simulink model "CruiseControl_PartialCoverageValid_harness"  (R2015a)
settings: Solver=FixedStepDiscrete  StartTime=0.0  StopTime=2  FixedStep=0.1  RelTol=1e-3
model workspace (MAT data in the model file):
  AccelResSw = mpt.Signal
  AccelResSw.DataType = 'boolean'
  AccelResSw.Min = 0
  AccelResSw.Max = 1
  AccelResSw.Dimensions = 1
  AccelResSw.DimensionsMode = 'Fixed'
  AccelResSw.Complexity = 'auto'
  AccelResSw.SampleTime = -1
  AccelResSw.SamplingMode = 'auto'
  Brake = mpt.Signal
  Brake.DataType = 'boolean'
  Brake.Min = 0
  Brake.Max = 1
  Brake.Dimensions = 1
  Brake.DimensionsMode = 'Fixed'
  Brake.Complexity = 'auto'
  Brake.SampleTime = -1
  Brake.SamplingMode = 'auto'
  CoastSetSw = mpt.Signal
  CoastSetSw.DataType = 'boolean'
  CoastSetSw.Min = 0
  CoastSetSw.Max = 1
  CoastSetSw.Dimensions = 1
  CoastSetSw.DimensionsMode = 'Fixed'
  CoastSetSw.Complexity = 'auto'
  CoastSetSw.SampleTime = -1
  CoastSetSw.SamplingMode = 'auto'
  CruiseOnOff = mpt.Signal
  CruiseOnOff.DataType = 'boolean'
  CruiseOnOff.Min = 0
  CruiseOnOff.Max = 1
  CruiseOnOff.Dimensions = 1
  CruiseOnOff.DimensionsMode = 'Fixed'
  CruiseOnOff.Complexity = 'auto'
  CruiseOnOff.SampleTime = -1
  CruiseOnOff.SamplingMode = 'auto'
  Speed = mpt.Signal
  Speed.DataType = 'uint8'
  Speed.Min = 0
  Speed.Max = 160
  Speed.Dimensions = 1
  Speed.DimensionsMode = 'Fixed'
  Speed.Complexity = 'auto'
  Speed.SampleTime = -1
  Speed.SamplingMode = 'auto'
  engaged = mpt.Signal
  engaged.DataType = 'boolean'
  engaged.Min = 0
  engaged.Max = 1
  engaged.Dimensions = 1
  engaged.DimensionsMode = 'Fixed'
  engaged.Complexity = 'auto'
  engaged.SampleTime = -1
  engaged.SamplingMode = 'auto'
  holdrate = mpt.Parameter
  holdrate.Value = 5
  holdrate.DataType = 'uint8'
  holdrate.Min = 1
  holdrate.Max = 10
  incdec = mpt.Parameter
  incdec.Value = 1
  incdec.DataType = 'uint8'
  incdec.Min = 1
  incdec.Max = 2
  maxtspeed = mpt.Parameter
  maxtspeed.Value = 90
  maxtspeed.DataType = 'uint8'
  maxtspeed.Min = 80
  maxtspeed.Max = 90
  mintspeed = mpt.Parameter
  mintspeed.Value = 20
  mintspeed.DataType = 'uint8'
  mintspeed.Min = 20
  mintspeed.Max = 25
  tspeed = mpt.Signal
  tspeed.DataType = 'uint8'
  tspeed.Min = 0
  tspeed.Max = 160
  tspeed.Dimensions = 1
  tspeed.DimensionsMode = 'Fixed'
  tspeed.Complexity = 'auto'
  tspeed.SampleTime = -1
  tspeed.SamplingMode = 'auto'
undefined symbols (not defined in the file or in its folder): sigbuilder_block
settings Model: PauseTimes=1.5  CovMetricSettings=dcmw  CovHTMLOptions=-sRT=1 -sVT=0 -aTS=0 -bRG=1 -bTC=1 -hTR=0 -nFC=0 -scm=1 -bcm=1 -xEv=0  CovSaveSingleToWorkspaceVar=off  CovCumulativeReport=on  CovReportOnPause=off  CovModelRefEnable=all  CovSFcnEnable=off  Creator=colosky  LastModifiedBy=colosky
settings DataIOCC: InspectSignalLogs=on
settings DebuggingCC: UnderspecifiedInitializationDetection=Classic  MergeDetectMultiDrivingBlocksExec=none  SolverPrmCheckMsg=warning

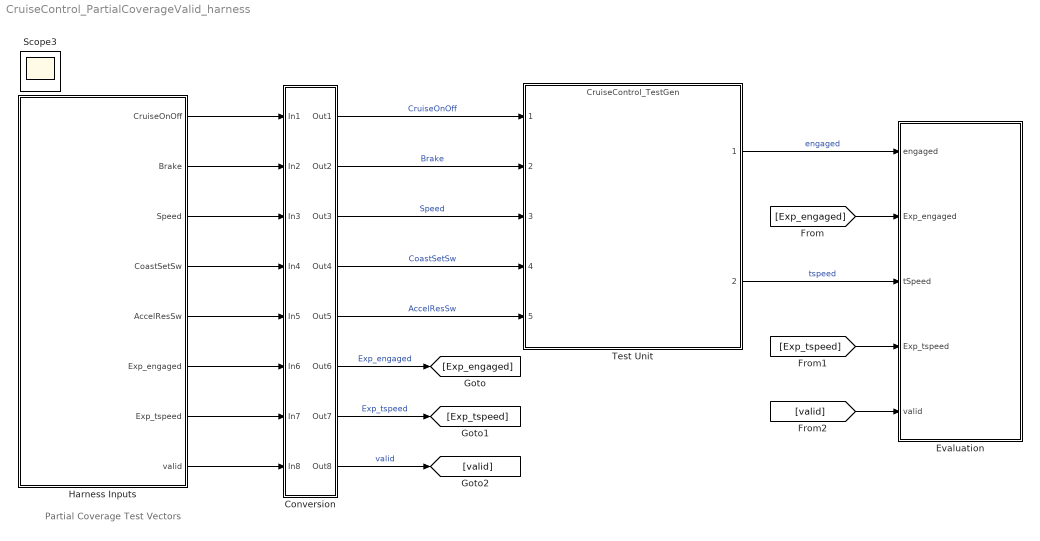
== system CruiseControl_PartialCoverageValid_harness ==
  note: Partial Coverage Test Vectors
  Conversion : Subsystem
      mask Display: disp(['Data' char(10) 'Type' char(10) 'Conv']);
  Evaluation : Subsystem
  Harness Inputs : Subsystem  Tag=STV Subsys  LoadFcn=sigbuilder_block('load',[756.6 77.4 520.2 400.2 ]);  StartFcn=sigbuilder_block('start');  StopFcn=sigbuilder_block('stop');  ClipboardFcn=sigbuilder_block('clipboard');  mask(Sigbuilder block){}
      mask init:
      | if ~strcmp(get_param(bdroot(gcb),'SimulationStatus'),'stopped'),tuvar = sigbuilder_block('maskInit'); end
      settings: CopyFcn=sigbuilder_block('copy');  DeleteFcn=sigbuilder_block('delete');  ModelCloseFcn=sigbuilder_block('modelClose');  PreSaveFcn=sigbuilder_block('preSave');  PauseFcn=sigbuilder_block('pause');  ContinueFcn=sigbuilder_block('continue');  NameChangeFcn=sigbuilder_block('namechange');  OpenFcn=sigbuilder_block('open');  CloseFcn=sigbuilder_block('close');
      mask Display: plot(0, 0, 100, 100,[2, 2, 32, 32, 2], [68, 8, 8, 68, 68],[32, 2], [38, 38], [32, 19, 2],[53, 60, 44], [32, 17, 17, 2],[16, 16, 31, 31]);txt = getActiveGroup(gcbh);text(2, 100, txt,'verticalAlignment', 'top');
  Test Unit : ModelReference  ModelNameDialog=CruiseControl_TestGen.slx  SimulationMode=Normal  ModelReferenceVersion=1.449  CopyOfModelName=CruiseControl_TestGen.slx  DefaultDataLogging=on
  Scope3 : Scope
      settings: SaveName=ScopeData3  MaxDataPoints=7500
  wires:
  Conversion/1(Out1) -> Test Unit/1  "CruiseOnOff"
  Conversion/5(Out5) -> Test Unit/5  "AccelResSw"
  Conversion/2(Out2) -> Test Unit/2  "Brake"
  Conversion/4(Out4) -> Test Unit/4  "CoastSetSw"
  Conversion/3(Out3) -> Test Unit/3  "Speed"
  Conversion/6(Out6) -> [Exp_engaged]  "Exp_engaged"
  Conversion/7(Out7) -> [Exp_tspeed]  "Exp_tspeed"
  Test Unit/1 -> Evaluation/1(engaged)  "engaged"
  Test Unit/2 -> Evaluation/3(tSpeed)  "tspeed"
  [Exp_engaged] -> Evaluation/2(Exp_engaged)
  [Exp_tspeed] -> Evaluation/4(Exp_tspeed)
  Harness Inputs/2(Brake) -> Conversion/2(In2)
  Harness Inputs/3(Speed) -> Conversion/3(In3)
  Harness Inputs/1(CruiseOnOff) -> Conversion/1(In1)
  Harness Inputs/4(CoastSetSw) -> Conversion/4(In4)
  Harness Inputs/5(AccelResSw) -> Conversion/5(In5)
  Harness Inputs/6(Exp_engaged) -> Conversion/6(In6)
  Harness Inputs/7(Exp_tspeed) -> Conversion/7(In7)
  Harness Inputs/8(valid) -> Conversion/8(In8)
  Conversion/8(Out8) -> [valid]  "valid"
  [valid] -> Evaluation/5(valid)

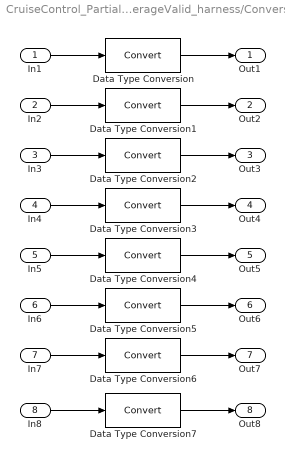
== system CruiseControl_PartialCoverageValid_harness/Conversion ==
  In1 : Inport
  In2 : Inport  Port=2
  In3 : Inport  Port=3
  In4 : Inport  Port=4
  In5 : Inport  Port=5
  In6 : Inport  Port=6
  In7 : Inport  Port=7
  In8 : Inport  Port=8
  Data Type Conversion{,1..7} (8 alike) : DataTypeConversion
  Out1 : Outport
  Out2 : Outport  Port=2
  Out3 : Outport  Port=3
  Out4 : Outport  Port=4
  Out5 : Outport  Port=5
  Out6 : Outport  Port=6
  Out7 : Outport  Port=7
  Out8 : Outport  Port=8
  wires:
  Data Type Conversion7/1 -> Out8/1
  In8/1 -> Data Type Conversion7/1
  In4/1 -> Data Type Conversion3/1
  Data Type Conversion4/1 -> Out5/1
  Data Type Conversion1/1 -> Out2/1
  In1/1 -> Data Type Conversion/1
  Data Type Conversion/1 -> Out1/1
  Data Type Conversion5/1 -> Out6/1
  In6/1 -> Data Type Conversion5/1
  Data Type Conversion6/1 -> Out7/1
  In7/1 -> Data Type Conversion6/1
  In5/1 -> Data Type Conversion4/1
  In2/1 -> Data Type Conversion1/1
  Data Type Conversion3/1 -> Out4/1
  In3/1 -> Data Type Conversion2/1
  Data Type Conversion2/1 -> Out3/1

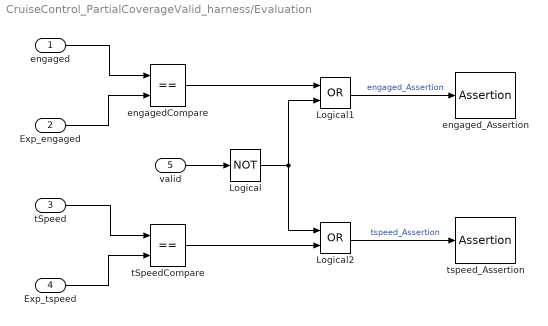
== system CruiseControl_PartialCoverageValid_harness/Evaluation ==
  engaged : Inport
  Exp_engaged : Inport  Port=2
  tSpeed : Inport  Port=3
  Exp_tspeed : Inport  Port=4
  valid : Inport  Port=5
  Logical : Logic  Operator=NOT  OutDataTypeStr=boolean
  Logical1 : Logic  Operator=OR  OutDataTypeStr=boolean
  Logical2 : Logic  Operator=OR  OutDataTypeStr=boolean
  engagedCompare : RelationalOperator  Operator===  OutDataTypeStr=boolean  InputSameDT=on
  engaged_Assertion : Assertion
  tSpeedCompare : RelationalOperator  Operator===  OutDataTypeStr=boolean  InputSameDT=on
  tspeed_Assertion : Assertion
  wires:
  Exp_engaged/1 -> engagedCompare/2
  engaged/1 -> engagedCompare/1
  Exp_tspeed/1 -> tSpeedCompare/2
  tSpeed/1 -> tSpeedCompare/1
  engagedCompare/1 -> Logical1/1
  tSpeedCompare/1 -> Logical2/2
  valid/1 -> Logical/1
  Logical1/1 -> engaged_Assertion/1  "engaged_Assertion"
  Logical/1 -> Logical2/1, Logical1/2
  Logical2/1 -> tspeed_Assertion/1  "tspeed_Assertion"

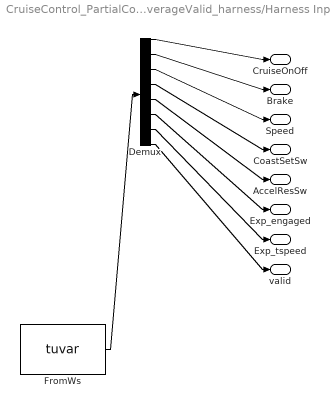
== system CruiseControl_PartialCoverageValid_harness/Harness Inputs ==
  Demux : Demux  Tag=STV Demux  Outputs=8
  FromWs : FromWorkspace  Tag=STV FromWs  VariableName=tuvar  SampleTime=0
      SigBuilderData=|
      | dataSet(1).timeRange = [0 2]
      | dataSet(1).name = 'Init Not Enable or Engaged'
      | dataSet(2).timeRange = [0 2]
      | dataSet(2).name = 'Not Engaged with Enable'
      | dataSet(3).timeRange = [0 2]
      | dataSet(3).name = 'Disengage with Disable'
      | dataSet(4).timeRange = [0 2]
      | dataSet(4).name = 'Engage 1st with CoastSetSW'
      | dataSet(5).timeRange = [0 2]
      | dataSet(5).name = 'No Engage 1st with AccelResSW'
      | dataSet(6).timeRange = [0 2]
      | dataSet(6).name = 'Disengage with Brake'
      | dataSet(7).timeRange = [0 2]
      | dataSet(7).name = 'Re-Engage with CoastSetSw'
      | dataSet(8).timeRange = [0 2]
      | dataSet(8).name = 'Re-Engage with AccelResSw'
      | dataSet(9).timeRange = [0 2]
      | dataSet(9).name = 'Engaged Decel with CoastSetSW'
      | dataSet(10).timeRange = [0 2]
      | dataSet(10).name = 'Engaged Accel with AccelResSW '
      | dataSet(11).timeRange = [0 2]
      | dataSet(11).name = 'Engagd Decel with CoastSet Hold'
      | dataSet(12).timeRange = [0 2]
      | dataSet(12).name = 'Engagd Accel with AccelRes Hold'
      | dataSet(13).timeRange = [0 2]
      | dataSet(13).name = 'Engage CoastSetSw Veh Spd'
      | dataSet(14).timeRange = [0 2]
      | dataSet(14).name = 'Engage AccelResSw Veh Spd '
      | sbobj.Name = 'Signal Builder'
      | sbobj.Groups(1).Name = 'Init Not Enable or Engaged'
      | sbobj.Groups(1).Signals(1).Name = 'CruiseOnOff'
      | sbobj.Groups(1).Signals(1).XData = [0 1 2]
      | sbobj.Groups(1).Signals(1).YData = [0 0 0]
      | sbobj.Groups(1).Signals(2).Name = 'Brake'
      | sbobj.Groups(1).Signals(2).XData = [0 1 2]
      | sbobj.Groups(1).Signals(2).YData = [0 0 0]
      | sbobj.Groups(1).Signals(3).Name = 'Speed'
      | sbobj.Groups(1).Signals(3).XData = [0 1 2]
      | sbobj.Groups(1).Signals(3).YData = [50 50 50]
      | sbobj.Groups(1).Signals(4).Name = 'CoastSetSw'
      | sbobj.Groups(1).Signals(4).XData = [0 1 2]
      | sbobj.Groups(1).Signals(4).YData = [0 0 0]
      | sbobj.Groups(1).Signals(5).Name = 'AccelResSw'
      | sbobj.Groups(1).Signals(5).XData = [0 1 2]
      | sbobj.Groups(1).Signals(5).YData = [0 0 0]
      | sbobj.Groups(1).Signals(6).Name = 'Exp_engaged'
      | sbobj.Groups(1).Signals(6).XData = [0 1 2]
      | sbobj.Groups(1).Signals(6).YData = [0 0 0]
      | sbobj.Groups(1).Signals(7).Name = 'Exp_tspeed'
      | sbobj.Groups(1).Signals(7).XData = [0 1 2]
      | sbobj.Groups(1).Signals(7).YData = [0 0 0]
      | sbobj.Groups(1).Signals(8).Name = 'valid'
      | sbobj.Groups(1).Signals(8).XData = [0 2]
      | sbobj.Groups(1).Signals(8).YData = [1 1]
      | sbobj.Groups(1).TimeRange = [0 2]
      | sbobj.Groups(2).Name = 'Not Engaged with Enable'
      | sbobj.Groups(2).Signals(1).Name = 'CruiseOnOff'
      | sbobj.Groups(2).Signals(1).XData = [0 1 1 1.5 1.5 2]
      | sbobj.Groups(2).Signals(1).YData = [0 0 1 1 0 0]
      | sbobj.Groups(2).Signals(2).Name = 'Brake'
      | sbobj.Groups(2).Signals(2).XData = [0 1 1.5 2]
      | sbobj.Groups(2).Signals(2).YData = [0 0 0 0]
      | sbobj.Groups(2).Signals(3).Name = 'Speed'
      | sbobj.Groups(2).Signals(3).XData = [0 1 1.5 2]
      | sbobj.Groups(2).Signals(3).YData = [0 0 0 0]
      | sbobj.Groups(2).Signals(4).Name = 'CoastSetSw'
      | sbobj.Groups(2).Signals(4).XData = [0 1 1.5 2]
      | sbobj.Groups(2).Signals(4).YData = [0 0 0 0]
      | sbobj.Groups(2).Signals(5).Name = 'AccelResSw'
      | sbobj.Groups(2).Signals(5).XData = [0 1 1.5 2]
      | sbobj.Groups(2).Signals(5).YData = [0 0 0 0]
      | sbobj.Groups(2).Signals(6).Name = 'Exp_engaged'
      | sbobj.Groups(2).Signals(6).XData = [0 1 1.5 2]
      | sbobj.Groups(2).Signals(6).YData = [0 0 0 0]
      | sbobj.Groups(2).Signals(7).Name = 'Exp_tspeed'
      | sbobj.Groups(2).Signals(7).XData = [0 1 1.5 2]
      | sbobj.Groups(2).Signals(7).YData = [0 0 0 0]
      | sbobj.Groups(2).Signals(8).Name = 'valid'
      | sbobj.Groups(2).Signals(8).XData = [0 2]
      | sbobj.Groups(2).Signals(8).YData = [1 1]
      | sbobj.Groups(2).TimeRange = [0 2]
      | sbobj.Groups(3).Name = 'Disengage with Disable'
      | sbobj.Groups(3).Signals(1).Name = 'CruiseOnOff'
      | sbobj.Groups(3).Signals(1).XData = [0 0.5 0.5 1 1.1 1.5 1.5 2]
      | sbobj.Groups(3).Signals(1).YData = [0 0 1 1 1 1 0 0]
      | sbobj.Groups(3).Signals(2).Name = 'Brake'
      | sbobj.Groups(3).Signals(2).XData = [0 0.5 1 1.1 1.5 2]
      | sbobj.Groups(3).Signals(2).YData = [0 0 0 0 0 0]
      | sbobj.Groups(3).Signals(3).Name = 'Speed'
      | sbobj.Groups(3).Signals(3).XData = [0 0.5 1 1.1 1.5 2]
      | sbobj.Groups(3).Signals(3).YData = [50 50 50 50 50 50]
      | sbobj.Groups(3).Signals(4).Name = 'CoastSetSw'
      | sbobj.Groups(3).Signals(4).XData = [0 0.5 1 1 1.1 1.1 1.5 2]
      | sbobj.Groups(3).Signals(4).YData = [0 0 0 1 1 0 0 0]
      | sbobj.Groups(3).Signals(5).Name = 'AccelResSw'
      | sbobj.Groups(3).Signals(5).XData = [0 0.5 1 1.1 1.5 2]
      | sbobj.Groups(3).Signals(5).YData = [0 0 0 0 0 0]
      | sbobj.Groups(3).Signals(6).Name = 'Exp_engaged'
      | sbobj.Groups(3).Signals(6).XData = [0 0.5 1 1 1.1 1.5 1.5 2]
      | sbobj.Groups(3).Signals(6).YData = [0 0 0 1 1 1 0 0]
      | sbobj.Groups(3).Signals(7).Name = 'Exp_tspeed'
      | sbobj.Groups(3).Signals(7).XData = [0 0.5 1 1 1.1 1.5 1.5 2]
      | sbobj.Groups(3).Signals(7).YData = [0 0 0 50 50 50 0 0]
      | sbobj.Groups(3).Signals(8).Name = 'valid'
      | sbobj.Groups(3).Signals(8).XData = [0 2]
      | sbobj.Groups(3).Signals(8).YData = [1 1]
      | sbobj.Groups(3).TimeRange = [0 2]
      | sbobj.Groups(4).Name = 'Engage 1st with CoastSetSW'
      | sbobj.Groups(4).Signals(1).Name = 'CruiseOnOff'
      | sbobj.Groups(4).Signals(1).XData = [0 0.5 0.5 1 1.1 2]
      | sbobj.Groups(4).Signals(1).YData = [0 0 1 1 1 1]
      | sbobj.Groups(4).Signals(2).Name = 'Brake'
      | sbobj.Groups(4).Signals(2).XData = [0 0.5 1 1.1 2]
      | sbobj.Groups(4).Signals(2).YData = [0 0 0 0 0]
      | sbobj.Groups(4).Signals(3).Name = 'Speed'
      | sbobj.Groups(4).Signals(3).XData = [0 0.5 1 1.1 2]
      | sbobj.Groups(4).Signals(3).YData = [50 50 50 50 50]
      | sbobj.Groups(4).Signals(4).Name = 'CoastSetSw'
      | sbobj.Groups(4).Signals(4).XData = [0 0.5 1 1 1.1 1.1 2]
      | sbobj.Groups(4).Signals(4).YData = [0 0 0 1 1 0 0]
      | sbobj.Groups(4).Signals(5).Name = 'AccelResSw'
      | sbobj.Groups(4).Signals(5).XData = [0 0.5 1 1.1 2]
      | sbobj.Groups(4).Signals(5).YData = [0 0 0 0 0]
      | sbobj.Groups(4).Signals(6).Name = 'Exp_engaged'
      | sbobj.Groups(4).Signals(6).XData = [0 0.5 1 1 1.1 2]
      | sbobj.Groups(4).Signals(6).YData = [0 0 0 1 1 1]
      | sbobj.Groups(4).Signals(7).Name = 'Exp_tspeed'
      | sbobj.Groups(4).Signals(7).XData = [0 0.5 1 1 1.1 2]
      | sbobj.Groups(4).Signals(7).YData = [0 0 0 50 50 50]
      | sbobj.Groups(4).Signals(8).Name = 'valid'
      | sbobj.Groups(4).Signals(8).XData = [0 2]
      | sbobj.Groups(4).Signals(8).YData = [1 1]
      | sbobj.Groups(4).TimeRange = [0 2]
      | sbobj.Groups(5).Name = 'No Engage 1st with AccelResSW'
      | sbobj.Groups(5).Signals(1).Name = 'CruiseOnOff'
      | sbobj.Groups(5).Signals(1).XData = [0 0.5 0.5 1 1.1 2]
      | sbobj.Groups(5).Signals(1).YData = [0 0 1 1 1 1]
      | sbobj.Groups(5).Signals(2).Name = 'Brake'
      | sbobj.Groups(5).Signals(2).XData = [0 0.5 1 1.1 2]
      | sbobj.Groups(5).Signals(2).YData = [0 0 0 0 0]
      | sbobj.Groups(5).Signals(3).Name = 'Speed'
      | sbobj.Groups(5).Signals(3).XData = [0 0.5 1 1.1 2]
      | sbobj.Groups(5).Signals(3).YData = [50 50 50 50 50]
      | sbobj.Groups(5).Signals(4).Name = 'CoastSetSw'
      | sbobj.Groups(5).Signals(4).XData = [0 0.5 1 1.1 2]
      | sbobj.Groups(5).Signals(4).YData = [0 0 0 0 0]
      | sbobj.Groups(5).Signals(5).Name = 'AccelResSw'
      | sbobj.Groups(5).Signals(5).XData = [0 0.5 1 1 1.1 1.1 2]
      | sbobj.Groups(5).Signals(5).YData = [0 0 0 1 1 0 0]
      | sbobj.Groups(5).Signals(6).Name = 'Exp_engaged'
      | sbobj.Groups(5).Signals(6).XData = [0 0.5 1 1.1 2]
      | sbobj.Groups(5).Signals(6).YData = [0 0 0 0 0]
      | sbobj.Groups(5).Signals(7).Name = 'Exp_tspeed'
      | sbobj.Groups(5).Signals(7).XData = [0 0.5 1 1.1 2]
      | sbobj.Groups(5).Signals(7).YData = [0 0 0 0 0]
      | sbobj.Groups(5).Signals(8).Name = 'valid'
      | sbobj.Groups(5).Signals(8).XData = [0 2]
      | sbobj.Groups(5).Signals(8).YData = [1 1]
      | sbobj.Groups(5).TimeRange = [0 2]
      | sbobj.Groups(6).Name = 'Disengage with Brake'
      | sbobj.Groups(6).Signals(1).Name = 'CruiseOnOff'
      | sbobj.Groups(6).Signals(1).XData = [0 0.5 0.5 1 1.1 1.5 1.6 2]
      | sbobj.Groups(6).Signals(1).YData = [0 0 1 1 1 1 1 1]
      | sbobj.Groups(6).Signals(2).Name = 'Brake'
      | sbobj.Groups(6).Signals(2).XData = [0 0.5 1 1.1 1.5 1.5 1.6 1.6 2]
      | sbobj.Groups(6).Signals(2).YData = [0 0 0 0 0 1 1 0 0]
      | sbobj.Groups(6).Signals(3).Name = 'Speed'
      | sbobj.Groups(6).Signals(3).XData = [0 0.5 1 1.1 1.5 1.6 2]
      | sbobj.Groups(6).Signals(3).YData = [50 50 50 50 50 50 50]
      | sbobj.Groups(6).Signals(4).Name = 'CoastSetSw'
      | sbobj.Groups(6).Signals(4).XData = [0 0.5 1 1 1.1 1.1 1.5 1.6 2]
      | sbobj.Groups(6).Signals(4).YData = [0 0 0 1 1 0 0 0 0]
      | sbobj.Groups(6).Signals(5).Name = 'AccelResSw'
      | sbobj.Groups(6).Signals(5).XData = [0 0.5 1 1.1 1.5 1.6 2]
      | sbobj.Groups(6).Signals(5).YData = [0 0 0 0 0 0 0]
      | sbobj.Groups(6).Signals(6).Name = 'Exp_engaged'
      | sbobj.Groups(6).Signals(6).XData = [0 0.5 1 1 1.1 1.5 1.5 1.6 2]
      | sbobj.Groups(6).Signals(6).YData = [0 0 0 1 1 1 0 0 0]
      | sbobj.Groups(6).Signals(7).Name = 'Exp_tspeed'
      | sbobj.Groups(6).Signals(7).XData = [0 0.5 1 1 1.1 1.5 1.6 2]
      | sbobj.Groups(6).Signals(7).YData = [0 0 0 50 50 50 50 50]
      | sbobj.Groups(6).Signals(8).Name = 'valid'
      | sbobj.Groups(6).Signals(8).XData = [0 2]
      | sbobj.Groups(6).Signals(8).YData = [1 1]
      | sbobj.Groups(6).TimeRange = [0 2]
      | sbobj.Groups(7).Name = 'Re-Engage with CoastSetSw'
      | sbobj.Groups(7).Signals(1).Name = 'CruiseOnOff'
      | sbobj.Groups(7).Signals(1).XData = [0 0.5 0.5 1 1.1 1.3 1.5 1.7 1.8 2]
      | sbobj.Groups(7).Signals(1).YData = [0 0 1 1 1 1 1 1 1 1]
      | sbobj.Groups(7).Signals(2).Name = 'Brake'
      | sbobj.Groups(7).Signals(2).XData = [0 0.5 1 1.1 1.3 1.3 1.5 1.5 1.7 1.8 2]
      | sbobj.Groups(7).Signals(2).YData = [0 0 0 0 0 1 1 0 0 0 0]
      | sbobj.Groups(7).Signals(3).Name = 'Speed'
      | sbobj.Groups(7).Signals(3).XData = [0 0.5 1 1.1 1.3 1.5 1.7 1.7 1.8 2]
      | sbobj.Groups(7).Signals(3).YData = [50 50 50 50 50 50 50 60 60 60]
      | sbobj.Groups(7).Signals(4).Name = 'CoastSetSw'
      | sbobj.Groups(7).Signals(4).XData = [0 0.5 1 1 1.1 1.1 1.3 1.5 1.7 1.7 1.8 1.8 2]
      | sbobj.Groups(7).Signals(4).YData = [0 0 0 1 1 0 0 0 0 1 1 0 0]
      | sbobj.Groups(7).Signals(5).Name = 'AccelResSw'
      | sbobj.Groups(7).Signals(5).XData = [0 0.5 1 1.1 1.3 1.5 1.7 1.8 2]
      | sbobj.Groups(7).Signals(5).YData = [0 0 0 0 0 0 0 0 0]
      | sbobj.Groups(7).Signals(6).Name = 'Exp_engaged'
      | sbobj.Groups(7).Signals(6).XData = [0 0.5 1 1 1.1 1.3 1.3 1.5 1.7 1.7 1.8 2]
      | sbobj.Groups(7).Signals(6).YData = [0 0 0 1 1 1 0 0 0 1 1 1]
      | sbobj.Groups(7).Signals(7).Name = 'Exp_tspeed'
      | sbobj.Groups(7).Signals(7).XData = [0 0.5 1 1 1.1 1.3 1.5 1.7 1.7 1.8 2]
      | sbobj.Groups(7).Signals(7).YData = [0 0 0 50 50 50 50 50 60 60 60]
      | sbobj.Groups(7).Signals(8).Name = 'valid'
      | sbobj.Groups(7).Signals(8).XData = [0 2]
      | sbobj.Groups(7).Signals(8).YData = [1 1]
      | sbobj.Groups(7).TimeRange = [0 2]
      | sbobj.Groups(8).Name = 'Re-Engage with AccelResSw'
      | sbobj.Groups(8).Signals(1).Name = 'CruiseOnOff'
      | sbobj.Groups(8).Signals(1).XData = [0 0.5 0.5 1 1.1 1.3 1.5 1.7 1.8 2]
      | sbobj.Groups(8).Signals(1).YData = [0 0 1 1 1 1 1 1 1 1]
      | sbobj.Groups(8).Signals(2).Name = 'Brake'
      | sbobj.Groups(8).Signals(2).XData = [0 0.5 1 1.1 1.3 1.3 1.5 1.5 1.7 1.8 2]
      | sbobj.Groups(8).Signals(2).YData = [0 0 0 0 0 1 1 0 0 0 0]
      | sbobj.Groups(8).Signals(3).Name = 'Speed'
      | sbobj.Groups(8).Signals(3).XData = [0 0.5 1 1.1 1.3 1.5 1.7 1.7 1.8 2]
      | sbobj.Groups(8).Signals(3).YData = [50 50 50 50 50 50 50 60 60 60]
      | sbobj.Groups(8).Signals(4).Name = 'CoastSetSw'
      | sbobj.Groups(8).Signals(4).XData = [0 0.5 1 1 1.1 1.1 1.3 1.5 1.7 1.8 2]
      | sbobj.Groups(8).Signals(4).YData = [0 0 0 1 1 0 0 0 0 0 0]
      | sbobj.Groups(8).Signals(5).Name = 'AccelResSw'
      | sbobj.Groups(8).Signals(5).XData = [0 0.5 1 1.1 1.3 1.5 1.7 1.7 1.8 1.8 2]
      | sbobj.Groups(8).Signals(5).YData = [0 0 0 0 0 0 0 1 1 0 0]
      | sbobj.Groups(8).Signals(6).Name = 'Exp_engaged'
      | sbobj.Groups(8).Signals(6).XData = [0 0.5 1 1 1.1 1.3 1.3 1.5 1.7 1.7 1.8 2]
      | sbobj.Groups(8).Signals(6).YData = [0 0 0 1 1 1 0 0 0 1 1 1]
      | sbobj.Groups(8).Signals(7).Name = 'Exp_tspeed'
      | sbobj.Groups(8).Signals(7).XData = [0 0.5 1 1 1.1 1.3 1.5 1.7 1.8 2]
      | sbobj.Groups(8).Signals(7).YData = [0 0 0 50 50 50 50 50 50 50]
      | sbobj.Groups(8).Signals(8).Name = 'valid'
      | sbobj.Groups(8).Signals(8).XData = [0 2]
      | sbobj.Groups(8).Signals(8).YData = [1 1]
      | sbobj.Groups(8).TimeRange = [0 2]
      | sbobj.Groups(9).Name = 'Engaged Decel with CoastSetSW'
      | sbobj.Groups(9).Signals(1).Name = 'CruiseOnOff'
      | sbobj.Groups(9).Signals(1).XData = [0 0.5 0.5 1 1.1 1.5 1.6 1.7 1.8 2]
      | sbobj.Groups(9).Signals(1).YData = [0 0 1 1 1 1 1 1 1 1]
      | sbobj.Groups(9).Signals(2).Name = 'Brake'
      | sbobj.Groups(9).Signals(2).XData = [0 0.5 1 1.1 1.5 1.6 1.7 1.8 2]
      | sbobj.Groups(9).Signals(2).YData = [0 0 0 0 0 0 0 0 0]
      | sbobj.Groups(9).Signals(3).Name = 'Speed'
      | sbobj.Groups(9).Signals(3).XData = [0 0.5 1 1.1 1.5 1.6 1.7 1.8 2]
      | sbobj.Groups(9).Signals(3).YData = [50 50 50 50 50 50 50 50 50]
      | sbobj.Groups(9).Signals(4).Name = 'CoastSetSw'
      | sbobj.Groups(9).Signals(4).XData = [0 0.5 1 1 1.1 1.1 1.5 1.5 1.6 1.6 1.7 1.7 1.8 1.8 2]
      | sbobj.Groups(9).Signals(4).YData = [0 0 0 1 1 0 0 1 1 0 0 1 1 0 0]
      | sbobj.Groups(9).Signals(5).Name = 'AccelResSw'
      | sbobj.Groups(9).Signals(5).XData = [0 0.5 1 1.1 1.5 1.6 1.7 1.8 2]
      | sbobj.Groups(9).Signals(5).YData = [0 0 0 0 0 0 0 0 0]
      | sbobj.Groups(9).Signals(6).Name = 'Exp_engaged'
      | sbobj.Groups(9).Signals(6).XData = [0 0.5 1 1 1.1 1.5 1.6 1.7 1.8 2]
      | sbobj.Groups(9).Signals(6).YData = [0 0 0 1 1 1 1 1 1 1]
      | sbobj.Groups(9).Signals(7).Name = 'Exp_tspeed'
      | sbobj.Groups(9).Signals(7).XData = [0 0.5 1 1 1.1 1.5 1.5 1.6 1.7 1.7 1.8 2]
      | sbobj.Groups(9).Signals(7).YData = [0 0 0 50 50 50 49 49 49 48 48 48]
      | sbobj.Groups(9).Signals(8).Name = 'valid'
      | sbobj.Groups(9).Signals(8).XData = [0 2]
      | sbobj.Groups(9).Signals(8).YData = [1 1]
      | sbobj.Groups(9).TimeRange = [0 2]
      | sbobj.Groups(10).Name = 'Engaged Accel with AccelResSW '
      | sbobj.Groups(10).Signals(1).Name = 'CruiseOnOff'
      | sbobj.Groups(10).Signals(1).XData = [0 0.5 0.5 1 1.1 1.5 1.6 1.7 1.8 2]
      | sbobj.Groups(10).Signals(1).YData = [0 0 1 1 1 1 1 1 1 1]
      | sbobj.Groups(10).Signals(2).Name = 'Brake'
      | sbobj.Groups(10).Signals(2).XData = [0 0.5 1 1.1 1.5 1.6 1.7 1.8 2]
      | sbobj.Groups(10).Signals(2).YData = [0 0 0 0 0 0 0 0 0]
      | sbobj.Groups(10).Signals(3).Name = 'Speed'
      | sbobj.Groups(10).Signals(3).XData = [0 0.5 1 1.1 1.5 1.6 1.7 1.8 2]
      | sbobj.Groups(10).Signals(3).YData = [50 50 50 50 50 50 50 50 50]
      | sbobj.Groups(10).Signals(4).Name = 'CoastSetSw'
      | sbobj.Groups(10).Signals(4).XData = [0 0.5 1 1 1.1 1.1 1.5 1.6 1.7 1.8 2]
      | sbobj.Groups(10).Signals(4).YData = [0 0 0 1 1 0 0 0 0 0 0]
      | sbobj.Groups(10).Signals(5).Name = 'AccelResSw'
      | sbobj.Groups(10).Signals(5).XData = [0 0.5 1 1.1 1.5 1.5 1.6 1.6 1.7 1.7 1.8 1.8 2]
      | sbobj.Groups(10).Signals(5).YData = [0 0 0 0 0 1 1 0 0 1 1 0 0]
      | sbobj.Groups(10).Signals(6).Name = 'Exp_engaged'
      | sbobj.Groups(10).Signals(6).XData = [0 0.5 1 1 1.1 1.5 1.6 1.7 1.8 2]
      | sbobj.Groups(10).Signals(6).YData = [0 0 0 1 1 1 1 1 1 1]
      | sbobj.Groups(10).Signals(7).Name = 'Exp_tspeed'
      | sbobj.Groups(10).Signals(7).XData = [0 0.5 1 1 1.1 1.5 1.5 1.6 1.7 1.7 1.8 2]
      | sbobj.Groups(10).Signals(7).YData = [0 0 0 50 50 50 51 51 51 52 52 52]
      | sbobj.Groups(10).Signals(8).Name = 'valid'
      | sbobj.Groups(10).Signals(8).XData = [0 2]
      | sbobj.Groups(10).Signals(8).YData = [1 1]
      | sbobj.Groups(10).TimeRange = [0 2]
      | sbobj.Groups(11).Name = 'Engagd Decel with CoastSet Hold'
      | sbobj.Groups(11).Signals(1).Name = 'CruiseOnOff'
      | sbobj.Groups(11).Signals(1).XData = [0 0.2 0.2 0.5 0.6 1 1.1 1.3 1.5 1.7 1.8 2]
      | sbobj.Groups(11).Signals(1).YData = [0 0 1 1 1 1 1 1 1 1 1 1]
      | sbobj.Groups(11).Signals(2).Name = 'Brake'
      | sbobj.Groups(11).Signals(2).XData = [0 0.2 0.5 0.6 1 1.1 1.3 1.5 1.7 1.8 2]
      | sbobj.Groups(11).Signals(2).YData = [0 0 0 0 0 0 0 0 0 0 0]
      | sbobj.Groups(11).Signals(3).Name = 'Speed'
      | sbobj.Groups(11).Signals(3).XData = [0 0.2 0.5 0.6 0.6 1 1.1 1.3 1.5 1.7 1.8 2]
      | sbobj.Groups(11).Signals(3).YData = [50 50 50 50 40 40 40 40 40 40 40 40]
      | sbobj.Groups(11).Signals(4).Name = 'CoastSetSw'
      | sbobj.Groups(11).Signals(4).XData = [0 0.2 0.5 0.5 0.6 0.6 1 1 1.1 1.1 1.3 1.3 1.5 1.7 1.8 1.8 2]
      | sbobj.Groups(11).Signals(4).YData = [0 0 0 1 1 0 0 1 1 0 0 1 1 1 1 0 0]
      | sbobj.Groups(11).Signals(5).Name = 'AccelResSw'
      | sbobj.Groups(11).Signals(5).XData = [0 0.2 0.5 0.6 1 1.1 1.3 1.5 1.7 1.8 2]
      | sbobj.Groups(11).Signals(5).YData = [0 0 0 0 0 0 0 0 0 0 0]
      | sbobj.Groups(11).Signals(6).Name = 'Exp_engaged'
      | sbobj.Groups(11).Signals(6).XData = [0 0.2 0.5 0.5 0.6 1 1.1 1.3 1.5 1.7 1.8 2]
      | sbobj.Groups(11).Signals(6).YData = [0 0 0 1 1 1 1 1 1 1 1 1]
      | sbobj.Groups(11).Signals(7).Name = 'Exp_tspeed'
      | sbobj.Groups(11).Signals(7).XData = [0 0.2 0.5 0.5 0.6 1 1 1.1 1.3 1.3 1.5 1.5 1.7 1.7 1.8 2]
      | sbobj.Groups(11).Signals(7).YData = [0 0 0 50 50 50 49 49 49 48 48 47 47 46 46 46]
      | sbobj.Groups(11).Signals(8).Name = 'valid'
      | sbobj.Groups(11).Signals(8).XData = [0 2]
      | sbobj.Groups(11).Signals(8).YData = [1 1]
      | sbobj.Groups(11).TimeRange = [0 2]
      | sbobj.Groups(12).Name = 'Engagd Accel with AccelRes Hold'
      | sbobj.Groups(12).Signals(1).Name = 'CruiseOnOff'
      | sbobj.Groups(12).Signals(1).XData = [0 0.2 0.2 0.5 0.6 1 1.1 1.3 1.5 1.7 1.8 2]
      | sbobj.Groups(12).Signals(1).YData = [0 0 1 1 1 1 1 1 1 1 1 1]
      | sbobj.Groups(12).Signals(2).Name = 'Brake'
      | sbobj.Groups(12).Signals(2).XData = [0 0.2 0.5 0.6 1 1.1 1.3 1.5 1.7 1.8 2]
      | sbobj.Groups(12).Signals(2).YData = [0 0 0 0 0 0 0 0 0 0 0]
      | sbobj.Groups(12).Signals(3).Name = 'Speed'
      | sbobj.Groups(12).Signals(3).XData = [0 0.2 0.5 0.6 0.6 1 1.1 1.3 1.5 1.7 1.8 2]
      | sbobj.Groups(12).Signals(3).YData = [50 50 50 50 40 40 40 40 40 40 40 40]
      | sbobj.Groups(12).Signals(4).Name = 'CoastSetSw'
      | sbobj.Groups(12).Signals(4).XData = [0 0.2 0.5 0.5 0.6 0.6 1 1.1 1.3 1.5 1.7 1.8 2]
      | sbobj.Groups(12).Signals(4).YData = [0 0 0 1 1 0 0 0 0 0 0 0 0]
      | sbobj.Groups(12).Signals(5).Name = 'AccelResSw'
      | sbobj.Groups(12).Signals(5).XData = [0 0.2 0.5 0.6 1 1 1.1 1.1 1.3 1.3 1.5 1.7 1.8 1.8 2]
      | sbobj.Groups(12).Signals(5).YData = [0 0 0 0 0 1 1 0 0 1 1 1 1 0 0]
      | sbobj.Groups(12).Signals(6).Name = 'Exp_engaged'
      | sbobj.Groups(12).Signals(6).XData = [0 0.2 0.5 0.5 0.6 1 1.1 1.3 1.5 1.7 1.8 2]
      | sbobj.Groups(12).Signals(6).YData = [0 0 0 1 1 1 1 1 1 1 1 1]
      | sbobj.Groups(12).Signals(7).Name = 'Exp_tspeed'
      | sbobj.Groups(12).Signals(7).XData = [0 0.2 0.5 0.5 0.6 1 1 1.1 1.3 1.3 1.5 1.5 1.7 1.7 1.8 2]
      | sbobj.Groups(12).Signals(7).YData = [0 0 0 50 50 50 51 51 51 52 52 53 53 54 54 54]
      | sbobj.Groups(12).Signals(8).Name = 'valid'
      | sbobj.Groups(12).Signals(8).XData = [0 2]
      | sbobj.Groups(12).Signals(8).YData = [1 1]
      | sbobj.Groups(12).TimeRange = [0 2]
      | sbobj.Groups(13).Name = 'Engage CoastSetSw Veh Spd'
      | sbobj.Groups(13).Signals(1).Name = 'CruiseOnOff'
      | sbobj.Groups(13).Signals(1).XData = [0 0.5 0.5 1 1.1 1.3 1.5 1.7 1.8 2]
      | sbobj.Groups(13).Signals(1).YData = [0 0 1 1 1 1 1 1 1 1]
      | sbobj.Groups(13).Signals(2).Name = 'Brake'
      | sbobj.Groups(13).Signals(2).XData = [0 0.5 1 1.1 1.3 1.5 1.7 1.8 2]
      | sbobj.Groups(13).Signals(2).YData = [0 0 0 0 0 0 0 0 0]
      | sbobj.Groups(13).Signals(3).Name = 'Speed'
      | sbobj.Groups(13).Signals(3).XData = [0 0.5 1 1.1 1.3 1.3 1.5 1.7 1.7 1.8 2]
      | sbobj.Groups(13).Signals(3).YData = [19 19 19 19 19 91 91 91 60 60 60]
      | sbobj.Groups(13).Signals(4).Name = 'CoastSetSw'
      | sbobj.Groups(13).Signals(4).XData = [0 0.5 1 1 1.1 1.1 1.3 1.3 1.5 1.5 1.7 1.7 1.8 1.8 2]
      | sbobj.Groups(13).Signals(4).YData = [0 0 0 1 1 0 0 1 1 0 0 1 1 0 0]
      | sbobj.Groups(13).Signals(5).Name = 'AccelResSw'
      | sbobj.Groups(13).Signals(5).XData = [0 0.5 1 1.1 1.3 1.5 1.7 1.8 2]
      | sbobj.Groups(13).Signals(5).YData = [0 0 0 0 0 0 0 0 0]
      | sbobj.Groups(13).Signals(6).Name = 'Exp_engaged'
      | sbobj.Groups(13).Signals(6).XData = [0 0.5 1 1.1 1.3 1.5 1.7 1.7 1.8 2]
      | sbobj.Groups(13).Signals(6).YData = [0 0 0 0 0 0 0 1 1 1]
      | sbobj.Groups(13).Signals(7).Name = 'Exp_tspeed'
      | sbobj.Groups(13).Signals(7).XData = [0 0.5 1 1.1 1.3 1.5 1.7 1.7 1.8 2]
      | sbobj.Groups(13).Signals(7).YData = [0 0 0 0 0 0 0 60 60 60]
      | sbobj.Groups(13).Signals(8).Name = 'valid'
      | sbobj.Groups(13).Signals(8).XData = [0 2]
      | sbobj.Groups(13).Signals(8).YData = [1 1]
      | sbobj.Groups(13).TimeRange = [0 2]
      | sbobj.Groups(14).Name = 'Engage AccelResSw Veh Spd '
      | sbobj.Groups(14).Signals(1).Name = 'CruiseOnOff'
      | sbobj.Groups(14).Signals(1).XData = [0 0.5 0.5 0.7 0.8 0.9 1 1.1 1.2 1.3 1.4 1.6 1.7 2]
      | sbobj.Groups(14).Signals(1).YData = [0 0 1 1 1 1 1 1 1 1 1 1 1 1]
      | sbobj.Groups(14).Signals(2).Name = 'Brake'
      | sbobj.Groups(14).Signals(2).XData = [0 0.5 0.7 0.8 0.9 0.9 1 1 1.1 1.2 1.3 1.4 1.6 1.7 2]
      | sbobj.Groups(14).Signals(2).YData = [0 0 0 0 0 1 1 0 0 0 0 0 0 0 0]
      | sbobj.Groups(14).Signals(3).Name = 'Speed'
      | sbobj.Groups(14).Signals(3).XData = [0 0.5 0.7 0.8 0.9 1 1.1 1.1 1.2 1.3 1.3 1.4 1.6 1.6 1.7 2]
      | sbobj.Groups(14).Signals(3).YData = [50 50 50 50 50 50 50 19 19 19 91 91 91 60 60 60]
      | sbobj.Groups(14).Signals(4).Name = 'CoastSetSw'
      | sbobj.Groups(14).Signals(4).XData = [0 0.5 0.7 0.7 0.8 0.8 0.9 1 1.1 1.2 1.3 1.4 1.6 1.7 2]
      | sbobj.Groups(14).Signals(4).YData = [0 0 0 1 1 0 0 0 0 0 0 0 0 0 0]
      | sbobj.Groups(14).Signals(5).Name = 'AccelResSw'
      | sbobj.Groups(14).Signals(5).XData = [0 0.5 0.7 0.8 0.9 1 1.1 1.1 1.2 1.2 1.3 1.3 1.4 1.4 1.6 1.6 1.7 1.7 2]
      | sbobj.Groups(14).Signals(5).YData = [0 0 0 0 0 0 0 1 1 0 0 1 1 0 0 1 1 0 0]
      | sbobj.Groups(14).Signals(6).Name = 'Exp_engaged'
      | sbobj.Groups(14).Signals(6).XData = [0 0.5 0.7 0.7 0.8 0.9 0.9 1 1.1 1.2 1.3 1.4 1.6 1.6 1.7 2]
      | sbobj.Groups(14).Signals(6).YData = [0 0 0 1 1 1 0 0 0 0 0 0 0 1 1 1]
      | sbobj.Groups(14).Signals(7).Name = 'Exp_tspeed'
      | sbobj.Groups(14).Signals(7).XData = [0 0.5 0.7 0.7 0.8 0.9 1 1.1 1.2 1.3 1.4 1.6 1.7 2]
      | sbobj.Groups(14).Signals(7).YData = [0 0 0 50 50 50 50 50 50 50 50 50 50 50]
      | sbobj.Groups(14).Signals(8).Name = 'valid'
      | sbobj.Groups(14).Signals(8).XData = [0 2]
      | sbobj.Groups(14).Signals(8).YData = [1 1]
      | sbobj.Groups(14).TimeRange = [0 2]
  CruiseOnOff : Outport
  Brake : Outport  Tag=STV Outport  Port=2
  Speed : Outport  Tag=STV Outport  Port=3
  CoastSetSw : Outport  Tag=STV Outport  Port=4
  AccelResSw : Outport  Tag=STV Outport  Port=5
  Exp_engaged : Outport  Tag=STV Outport  Port=6
  Exp_tspeed : Outport  Tag=STV Outport  Port=7
  valid : Outport  Tag=STV Outport  Port=8
  wires:
  FromWs/1 -> Demux/1
  Demux/1 -> CruiseOnOff/1
  Demux/2 -> Brake/1
  Demux/3 -> Speed/1
  Demux/4 -> CoastSetSw/1
  Demux/5 -> AccelResSw/1
  Demux/6 -> Exp_engaged/1
  Demux/7 -> Exp_tspeed/1
  Demux/8 -> valid/1
